simulink library "tqen"  (Simulink 8.2)
settings: Solver=ode45  SolverMode=SingleTasking  StartTime=0.0  StopTime=10.0  RelTol=1e-3
undefined symbols (not defined in the file or in its folder): ATQEN_BaseBrkDerateRatD_X_pct, ATQEN_BaseVehSpdRatD_X_kph, ATQEN_CruzAccLimIMult_X_mps2, ATQEN_CruzAccLimPMult_X_mps2, ATQEN_CruzContIMult_X_kph, ATQEN_CruzContPMult_X_kph, ATQEN_EngTqBrkMap_X_erpm, C_TASK_5MS_S, C_TICK_TIME_S, ENUM_ECMTQSOURCE_EXTERNAL, ENUM_ECMTQSOURCE_INTERNAL, ENUM_ECMTQSOURCE_TORQUELIM, ENUM_EMSHYBRIDOPSTATE_HYBRIDENABLE, ENUM_EMSOPSTATE_NORMAL, ENUM_GEARPOSN_PN, FALSE, KTQEN_AccelPedalFiltTm_s, KTQEN_BrakeSWTqDsblTimeThres_s, KTQEN_CruzAccLimErrGain_rat, KTQEN_CruzAccLimIGain_rat, KTQEN_CruzAccLimIMax_Nm, KTQEN_CruzAccLimIMin_Nm, KTQEN_CruzAccLimIRest_flg, KTQEN_CruzAccLimPGain_rat, KTQEN_CruzContAccLim_G, KTQEN_CruzContAccLimTqMax_Nm, KTQEN_CruzContAccLimTqMin_Nm, KTQEN_CruzContEnblSW_flg, KTQEN_CruzContErrGain_rat, KTQEN_CruzContIGain_rat, KTQEN_CruzContIMax_Nm, KTQEN_CruzContIMin_Nm, KTQEN_CruzContIRest_flg, KTQEN_CruzContPGain_rat, KTQEN_CruzContResumeSW_flg, KTQEN_CruzContSetSW_flg, KTQEN_CruzDsblDefaultTq_Nm, KTQEN_CruzSpdChgTimeThres_s, KTQEN_CruzTgSpdSetFalRate_kphps, KTQEN_CruzTgSpdSetRisRate_kphps, KTQEN_EngBrkTqMaxOvrd_Nm, KTQEN_EngBrkTqMinOvrd_Nm, KTQEN_VehAccCalRate_s, KTQEN_VehAccFltConst_s, KTQEN_VehSpdMaxVal_kph, KTQEN_VSGOVErrGain_rat, KTQEN_VSGOVIGain_rat, KTQEN_VSGOVIMax_Nm, KTQEN_VSGOVIMin_Nm, KTQEN_VSGOVIRest_flg, KTQEN_VSGOVMinVehSpd_kph, KTQEN_VSGOVPGain_rat, KTQEN_VSGOVTqDefault_Nm, KTQEN_VSGOVTqMax_Nm, KTQEN_VSGOVTqMin_Nm, MTQEN_BaseBrkDerateRatD_Y_pct, MTQEN_BasePedalSportMapHiSpdD_Z_pct, MTQEN_BasePedalSportMapLoSpdD_Z_pct, MTQEN_BaseTqSupptDeltPdlD_X_pctps, MTQEN_BaseTqSupptDeltPdlD_Y_pct ... (+9)
libraries: hcu_lib x6, tqen x3, simulink x1
(part 1 of 2)
settings Model: Creator=13192  LastModifiedBy=14069

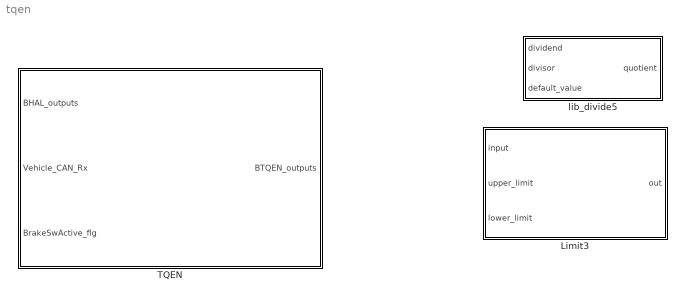
== system tqen ==
  Limit3 : Subsystem
      mask Display: disp('Limitation')
  TQEN : Subsystem
      settings: RTWSystemCode=Nonreusable function  RTWFcnNameOpts=Use subsystem name  RTWFileNameOpts=Use subsystem name
  lib_divide5 : Subsystem  RTWFcnName=plaus_check  mask(divide){}
      mask help: Performs a division operation. If the divisor is found to be between -0.00001 and +0.00001 then a failsafe value is passed to the output.
      mask Display: disp('Divide\nTQM');

== system tqen/Limit3 ==
  input : Inport
  upper_limit : Inport  Port=2
  lower_limit : Inport  Port=3
  MinMax10 : MinMax  Function=max  Inputs=2
  MinMax5 : MinMax  Inputs=2
  out : Outport
  wires:
  lower_limit/1 -> MinMax10/2
  upper_limit/1 -> MinMax5/2
  MinMax10/1 -> out/1
  input/1 -> MinMax5/1
  MinMax5/1 -> MinMax10/1

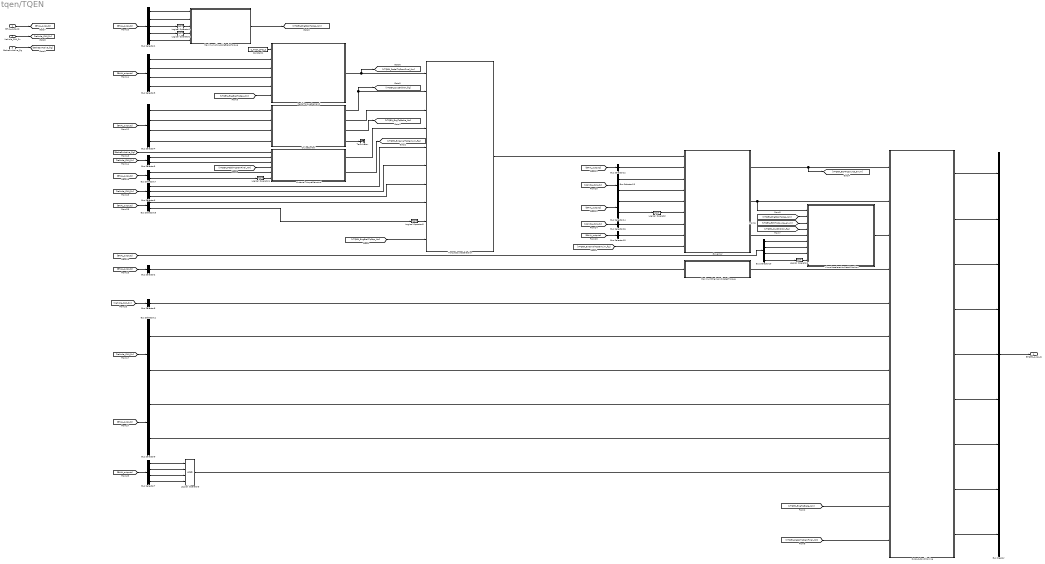
== system tqen/TQEN ==
  BHAL_outputs : Inport  OutDataTypeStr=Bus: BHAL_outputs
  Vehicle_CAN_Rx : Inport  Port=2
  BrakeSwActive_flg : Inport  Port=3
  Bus Creator : BusCreator  Inputs=9  OutDataTypeStr=Bus: BTQEN_outputs
  Bus Selector1 : BusSelector  OutputSignals=VHAL_EngTqMax_Nm,VHAL_EngTqMin_Nm,VHAL_EngTqMinInvalid_flg,VHAL_EngTqMaxInvalid_flg,VHAL_EngSpd_erpm
  Bus Selector10 : BusSelector  OutputSignals=VHAL_EngSpd_erpm,VHAL_AccelPedalPosn_pct,VHAL_EngTqMin_Nm,VHAL_EngTqMinInvalid_flg
  Bus Selector11 : BusSelector  OutputSignals=ADAS2.ADAS_PTTqReq,ADAS2.ADAS_PTTqReq_A
  Bus Selector12 : BusSelector  OutputSignals=VHAL_VehSpd_kph
  Bus Selector13 : BusSelector  OutputSignals=ADAS3.ADAS_VehSpdLim,ADAS3.ADAS_VehSpdLim_A
  Bus Selector14 : BusSelector  OutputSignals=VHAL_NowGearPosn_enum,VHAL_VehSpdInvalid_flg
  Bus Selector15 : BusSelector  OutputSignals=VHAL_BrkLampOn_flg
  Bus Selector16 : BusSelector  OutputSignals=ADAS2.ADAS_PTTqReq_A
  Bus Selector17 : BusSelector  OutputSignals=VHAL_EngTqMin_Nm,VHAL_EngTqMinInvalid_flg
  Bus Selector18 : BusSelector  OutputSignals=VHAL_EngTqMin_Nm,VHAL_EngTqMinInvalid_flg
  Bus Selector2 : BusSelector  OutputSignals=VHAL_EngTqFriction_Nm
  Bus Selector3 : BusSelector  OutputSignals=VHAL_AccelPedalPosn_pct,VHAL_BrkLampOn_flg,VHAL_EngSpd_erpm,VHAL_VehSpd_kph
  Bus Selector4 : BusSelector  OutputSignals=VHAL_BrkLampOn_flg,VHAL_VehSpd_kph,VHAL_EngTqIndicatedCOR_Nm,VHAL_EngTqFriction_Nm
  Bus Selector5 : BusSelector  OutputSignals=ADAS2.ADAS_PTTqReq,ADAS2.ADAS_PTTqReq_A
  Bus Selector6 : BusSelector  OutputSignals=ADAS2.ADAS_PTTqReq_A,ADAS2.ADAS_ForceIdle,ADAS2.ADAS_ForceIdle_A
  Bus Selector7 : BusSelector  OutputSignals=VHAL_CANMsgValidECM1_flg,VHAL_CANMsgValidECM2_flg,VHAL_CANMsgValidECM3_flg,VHAL_CANMsgValidECM9_flg
  Bus Selector8 : BusSelector  OutputSignals=ECM1.CAN_TQ_STND
  Bus Selector9 : BusSelector  OutputSignals=VHAL_EMSHybridOpState_enum,VHAL_EMSOpState_enum
  Constant1 : Constant  Value=C_TASK_5MS_S  OutDataTypeStr=single
  CruiseControl : Subsystem  TreatAsAtomicUnit=on
  ExternalTorqueDemand : Subsystem
  Governor : Subsystem
  Logical Operator{,1..2,4..6} (6 alike) : Logic  Operator=NOT  AllPortsSameDT=off  OutDataTypeStr=boolean
  Logical Operator3 : Logic  Inputs=4  AllPortsSameDT=off  OutDataTypeStr=boolean
  MaximumAllowableBrakeTorque : Subsystem
  MaximumEngineIndicatedTorque : Subsystem
  Output_Conditioning : Subsystem
  PedalTorqueDemand : Subsystem
  Terminator : Terminator
  TorqueSourceSelection : Subsystem
  VirtualAccelerationPedalPosition : Subsystem
  BTQEN_outputs : Outport  OutDataTypeStr=Bus: BTQEN_outputs
  wires:
  Logical Operator6/1 -> VirtualAccelerationPedalPosition/9(VDINR_EngTqMinValid_flg)
  Bus Selector10/4 -> Logical Operator6/1  "<VHAL_EngTqMinInvalid_flg>"
  Bus Selector10/3 -> VirtualAccelerationPedalPosition/8(VDINR_EngTqMin_Nm)  "<VHAL_EngTqMin_Nm>"
  Logical Operator5/1 -> TorqueSourceSelection/9(VDINR_EngTqMinValid_flg)
  [BHAL_outputs] -> Bus Selector18/1
  Bus Selector18/2 -> Logical Operator5/1  "<VHAL_EngTqMinInvalid_flg>"
  Bus Selector18/1 -> TorqueSourceSelection/8(VDINR_EngTqMin_Nm)  "<VHAL_EngTqMin_Nm>"
  Logical Operator4/1 -> ExternalTorqueDemand/6(VDINR_EngTqMinValid_flg)
  [BHAL_outputs] -> Bus Selector17/1
  Bus Selector17/2 -> Logical Operator4/1  "<VHAL_EngTqMinInvalid_flg>"
  Bus Selector17/1 -> ExternalTorqueDemand/5(VDINR_EngTqMin_Nm)  "<VHAL_EngTqMin_Nm>"
  [BHAL_outputs] -> Bus Selector9/1
  Logical Operator3/1 -> Output_Conditioning/10(VDINR_ECMCANValid_flg)
  Bus Selector7/2 -> Logical Operator3/2  "<VHAL_CANMsgValidECM2_flg>"
  Bus Selector7/4 -> Logical Operator3/4  "<VHAL_CANMsgValidECM9_flg>"
  Bus Selector7/3 -> Logical Operator3/3  "<VHAL_CANMsgValidECM3_flg>"
  Bus Selector7/1 -> Logical Operator3/1  "<VHAL_CANMsgValidECM1_flg>"
  [BHAL_outputs] -> Bus Selector7/1
  Bus Selector15/1 -> Governor/8(VDINR_BrkLampOn_flg)  "<VHAL_BrkLampOn_flg>"
  Bus Selector16/1 -> Governor/7(VDINR_ADASPTTqReqApplable_flg)  "<ADAS_PTTqReq_A>"
  [Vehicle_CAN_Rx] -> Bus Selector16/1
  [BHAL_outputs] -> Bus Selector15/1
  Bus Selector14/2 -> Logical Operator/1  "<VHAL_VehSpdInvalid_flg>"
  Bus Selector14/1 -> Governor/5(VDINR_NowGearPosn_enum)  "<VHAL_NowGearPosn_enum>"
  Bus Selector13/2 -> Governor/4(VDINR_ADASVehSpdLimReqValid_flg)  "<ADAS_VehSpdLim_A>"
  Bus Selector13/1 -> Governor/3(VDINR_ADASVehSpdLimReq_kph)  "<ADAS_VehSpdLim>"
  [BHAL_outputs] -> Bus Selector14/1
  [VTQEN_PedalTqDemFinal_Nm] -> ExternalTorqueDemand/4(VTQEN_PedalTqDemFinal_Nm)
  Output_Conditioning/9("VTQEN_PedalTqDemFinal_Nm ") -> Bus Creator/9
  [VTQEN_PedalTqDemFinal_Nm] -> Output_Conditioning/12(VTQEN_PedalTqDemFinal_Nm)
  Bus Selector6/3 -> TorqueSourceSelection/7(VDINR_ADASPTIdleReqValid_flg)  "<ADAS_ForceIdle_A>"
  Bus Selector6/2 -> TorqueSourceSelection/6(VDINR_ADASPTIdleReq_flg)  "<ADAS_ForceIdle>"
  Output_Conditioning/3("VTQEN_FinalAccelPedalPosn_pct ") -> Bus Creator/3
  Bus Selector10/2 -> VirtualAccelerationPedalPosition/7(VDINR_HWAccelPedalPosn_pct)  "<VHAL_AccelPedalPosn_pct>"
  Bus Selector10/1 -> VirtualAccelerationPedalPosition/6(VDINR_EngSpd_erpm)  "<VHAL_EngSpd_erpm>"
  [VTQEN_CruzEnblOn_flg] -> VirtualAccelerationPedalPosition/4(VTQEN_CruzEnblOn_flg)
  [VTQEN_ECMTqSource_enum] -> VirtualAccelerationPedalPosition/3(VTQEN_ECMTqSource_enum)
  [VTQEN_EngBrakTqCap_Nm] -> VirtualAccelerationPedalPosition/2(VTQEN_EngBrakTqCap_Nm)
  Governor/3(VTQEN_VSGOVOn_flg) -> VirtualAccelerationPedalPosition/5(VTQEN_VSGOVOn_flg)
  VirtualAccelerationPedalPosition/1(VTQEN_FinalAccelPedalPosn_pct) -> Output_Conditioning/3(VTQEN_FinalAccelPedalPosn_pct)
  [VTQEN_ExternalTqDemLim_flg] -> Governor/9(VTQEN_ExternalTqDemLim_flg)
  ExternalTorqueDemand/2(VTQEN_ExternalTqDemLim_flg) -> [VTQEN_ExternalTqDemLim_flg]
  Output_Conditioning/8("VTQEN_EngTqBrake_Nm ") -> Bus Creator/8
  Output_Conditioning/7(VTQEN_ECMExtnTqAvailable_flg) -> Bus Creator/7
  Output_Conditioning/6(VTQEN_AckCurPTTqReqApplable_flg) -> Bus Creator/6
  Output_Conditioning/5(VTQEN_AckCurPTTqReq_Nm) -> Bus Creator/5
  Bus Selector11/2 -> Output_Conditioning/7(VDINR_ADASPTTqReqApplable_flg)  "<ADAS_PTTqReq_A>"
  Bus Selector11/1 -> Output_Conditioning/6(VDINR_ADASPTTqReq_Nm)  "<ADAS_PTTqReq>"
  [VTQEN_EngTqBrake_Nm] -> Output_Conditioning/11(VTQEN_EngTqBrake_Nm)
  Output_Conditioning/1("VTQEN_ECMTqSource_enum ") -> Bus Creator/1
  CruiseControl/3(VTQEN_EngTqBrake_Nm) -> [VTQEN_EngTqBrake_Nm]
  Logical Operator/1 -> Governor/6(VDINR_VehSpdValid_flg)
  Governor/1(VTQEN_ECMTqSource_enum) -> [VTQEN_ECMTqSource_enum], Output_Conditioning/1(VTQEN_ECMTqSource_enum)
  Output_Conditioning/4(VTQEN_EngIndTqReqMax_pct) -> Bus Creator/4
  Output_Conditioning/2(VTQEN_EngBrakTqReqFinal_Nm) -> Bus Creator/2
  Governor/2(VTQEN_EngBrakTqReqFinal_Nm) -> VirtualAccelerationPedalPosition/1(VTQEN_EngBrakTqReqFinal_Nm), Output_Conditioning/2("VTQEN_EngBrakTqReqFinal_Nm ")
  MaximumEngineIndicatedTorque/1(VTQEN_EngIndTqReqMax_Nm) -> Output_Conditioning/4(VTQEN_EngIndTqReqMax_Nm)
  ExternalTorqueDemand/1(VTQEN_ExternalTqDem_Nm) -> TorqueSourceSelection/4(VTQEN_ExternalTqDem_Nm)
  CruiseControl/2(VTQEN_CruzContTqComdFinal_Nm) -> TorqueSourceSelection/3(VTQEN_CruzContTqComdFinal_Nm)
  CruiseControl/1(VTQEN_CruzEnblOn_flg) -> [VTQEN_CruzEnblOn_flg], TorqueSourceSelection/2(VTQEN_CruzEnblOn_flg)
  Bus Selector6/1 -> TorqueSourceSelection/5(VDINR_ADASPTTqReqApplable_flg)  "<ADAS_PTTqReq_A>"
  CruiseControl/4(VTQEN_CruzStandby_flg) -> Terminator/1
  Bus Selector4/4 -> CruiseControl/4(VDINR_EngTqFriction_Nm)  "<VHAL_EngTqFriction_Nm>"
  Bus Selector4/3 -> CruiseControl/3(VDINR_EngTqIndicatedCOR_Nm)  "<VHAL_EngTqIndicatedCOR_Nm>"
  Bus Selector4/2 -> CruiseControl/2(VDINR_VehSpd_kph)  "<VHAL_VehSpd_kph>"
  Bus Selector4/1 -> CruiseControl/1(VDINR_BrkLampOn_flg)  "<VHAL_BrkLampOn_flg>"
  [VTQEN_EngBrakTqCap_Nm] -> TorqueSourceSelection/10(VTQEN_EngBrakTqCap_Nm)
  [VTQEN_EngBrakTqCap_Nm] -> PedalTorqueDemand/6(VTQEN_EngBrakTqCap_Nm)
  Bus Creator/1 -> BTQEN_outputs/1  "BTQEN_outputs"
  [BHAL_outputs] -> Bus Selector1/1
  TorqueSourceSelection/1(VTQEN_EngBrakTqReqRaw_Nm) -> Governor/1(VTQEN_EngBrakTqReqRaw_Nm)
  MaximumAllowableBrakeTorque/1(VTQEN_EngBrakTqCap_Nm) -> [VTQEN_EngBrakTqCap_Nm]
  PedalTorqueDemand/1(VTQEN_PedalTqDemFinal_Nm) -> [VTQEN_PedalTqDemFinal_Nm], TorqueSourceSelection/1(VTQEN_PedalTqDemFinal_Nm)
  Bus Selector1/1 -> MaximumAllowableBrakeTorque/1(VDINR_EngTqMax_Nm)  "<VHAL_EngTqMax_Nm>"
  Bus Selector1/2 -> MaximumAllowableBrakeTorque/2(VDINR_EngTqMin_Nm)  "<VHAL_EngTqMin_Nm>"
  Bus Selector1/3 -> Logical Operator1/1  "<VHAL_EngTqMinInvalid_flg>"
  Bus Selector1/4 -> Logical Operator2/1  "<VHAL_EngTqMaxInvalid_flg>"
  Bus Selector1/5 -> MaximumAllowableBrakeTorque/5(VDINR_EngSpd_erpm)  "<VHAL_EngSpd_erpm>"
  Constant1/1 -> PedalTorqueDemand/1(task_time_s)
  Bus Selector8/1 -> Output_Conditioning/5(VDINR_StandardTq_Nm)  "<CAN_TQ_STND>"
  Bus Selector2/1 -> MaximumEngineIndicatedTorque/1(VDINR_EngTqFriction_Nm)  "<VHAL_EngTqFriction_Nm>"
  Logical Operator1/1 -> MaximumAllowableBrakeTorque/3(VDINR_EngTqMinValid_flg)
  Logical Operator2/1 -> MaximumAllowableBrakeTorque/4(VDINR_EngTqMaxValid_flg)
  Bus Selector3/4 -> PedalTorqueDemand/5(VDINR_VehSpd_kph)  "<VHAL_VehSpd_kph>"
  Bus Selector3/1 -> PedalTorqueDemand/2(VDINR_HWAccelPedalPosn_pct)  "<VHAL_AccelPedalPosn_pct>"
  Bus Selector3/2 -> PedalTorqueDemand/3(VDINR_BrkLampOn_flg)  "<VHAL_BrkLampOn_flg>"
  Bus Selector3/3 -> PedalTorqueDemand/4(VDINR_EngSpd_erpm)  "<VHAL_EngSpd_erpm>"
  [BrakeSwActive_flg] -> ExternalTorqueDemand/1(VDINR_BrakeSwActive_flg)
  [Vehicle_CAN_Rx] -> Bus Selector5/1
  Bus Selector5/2 -> ExternalTorqueDemand/3(VDINR_ADASPTTqReqValid_flg)  "<ADAS_PTTqReq_A>"
  Bus Selector5/1 -> ExternalTorqueDemand/2(VDINR_ADASPTTqReq_Nm)  "<ADAS_PTTqReq>"
  BHAL_outputs/1 -> [BHAL_outputs]
  Vehicle_CAN_Rx/1 -> [Vehicle_CAN_Rx]
  BrakeSwActive_flg/1 -> [BrakeSwActive_flg]
  [BHAL_outputs] -> Bus Selector3/1
  [BHAL_outputs] -> Bus Selector4/1
  [Vehicle_CAN_Rx] -> Bus Selector6/1
  [BHAL_outputs] -> Bus Selector2/1
  [Vehicle_CAN_Rx] -> Bus Selector11/1
  Bus Selector9/1 -> Output_Conditioning/8(VDINR_EMSHybridOpState_enum)  "<VHAL_EMSHybridOpState_enum>"
  Bus Selector9/2 -> Output_Conditioning/9(VDINR_EMSOpState_enum)  "<VHAL_EMSOpState_enum>"
  [Vehicle_CAN_Rx] -> Bus Selector8/1
  [BHAL_outputs] -> Bus Selector10/1
  [BHAL_outputs] -> Bus Selector12/1
  Bus Selector12/1 -> Governor/2(VDINR_VehSpd_kph)  "<VHAL_VehSpd_kph>"
  [Vehicle_CAN_Rx] -> Bus Selector13/1

== system tqen/lib_divide5 ==
  dividend : Inport
  divisor : Inport  Port=2
  default_value : Inport  Port=3
  Divide : Product  Inputs=*/
  Inter_Test : Subsystem  mask(Interval Test){IntervalClosedRight=on, uplimit=0.00001, IntervalClosedLeft=on, lowlimit=-0.00001, LogicOutDataTypeMode=boolean}
      mask prompts: IntervalClosedRight "Interval closed on right"; uplimit "Upper limit:"; IntervalClosedLeft "Interval closed on left"; lowlimit "Lower limit:"; LogicOutDataTypeMode "Output data type mode:"
      mask help: If the input is in the interval between the lower limit and the upper limit, then the output is TRUE, otherwise it is FALSE.
      mask init:
      | if IntervalClosedLeft
      |   lOff = 0;
      |   lRelop = '<=';
      | else
      |   lOff = 0.1;
      |   lRelop = '<';
      | end
      | if IntervalClosedRight
      |   rOff = 0;
      |   uRelop = '<=';
      | else
      |   rOff = 0.1;
      |   uRelop = '<';
      | end
      | 
      | blkH = gcbh;
      | blkName = getfullname(blkH);
      | 
      | set_param([blkName,'/Upper_Test'],'relop',uRelop);
      | set_param([blkName,'/Lower_Test'],'relop',lRelop);
      | if strcmp(get_param(blkH,'LogicOutDataTypeMode'),'boolean')
      | set_param([blkName,'/AND'],'OutDataTypeMode','Boolean');
      | else
      | set_param([blkName,'/AND'],'OutDataTypeMode','Specify via dialog');
      | end
      mask TypeOptions LogicOutDataTypeMode: uint8 | boolean
      mask Display: plot([0 1],[0.3 0.3],[0.3 0.3],[0 1],[0 0.2 0.2],[0.35 0.35 0.55-lOff],[0.2 0.2 0.55 0.55],[0.55+lOff 0.75 0.75 0.55+rOff],[0.55 0.55 1],[0.55-rOff 0.35 0.35]);
  Logical_Operator : Logic  Operator=NOT  AllPortsSameDT=off  OutDataTypeStr=boolean
  Switch : Switch  Criteria=u2 ~= 0  Threshold=0.5
  quotient : Outport
  wires:
  divisor/1 -> Inter_Test/1(u), Divide/2
  dividend/1 -> Divide/1
  Divide/1 -> Switch/1
  Switch/1 -> quotient/1
  Inter_Test/1(y) -> Logical_Operator/1
  default_value/1 -> Switch/3
  Logical_Operator/1 -> Switch/2

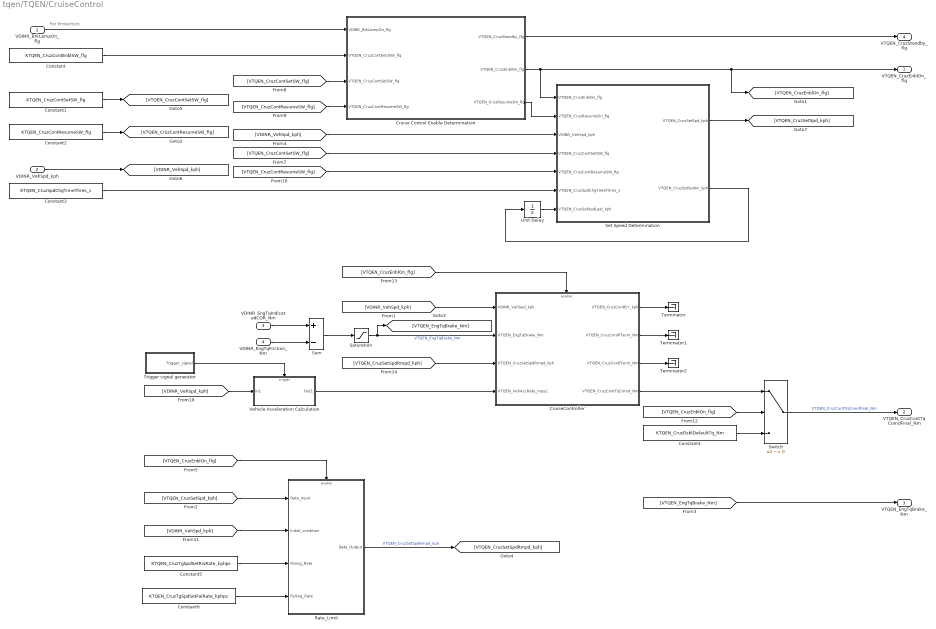
== system tqen/TQEN/CruiseControl ==
  note: For Protection
  VDINR_BrkLampOn_flg : Inport
  VDINR_VehSpd_kph : Inport  Port=2
  VDINR_EngTqIndicatedCOR_Nm : Inport  Port=3
  VDINR_EngTqFriction_Nm : Inport  Port=4
  Constant : Constant  Value=KTQEN_CruzContEnblSW_flg
  Constant1 : Constant  Value=KTQEN_CruzContSetSW_flg
  Constant2 : Constant  Value=KTQEN_CruzContResumeSW_flg
  Constant3 : Constant  Value=KTQEN_CruzSpdChgTimeThres_s
  Constant4 : Constant  Value=KTQEN_CruzDsblDefaultTq_Nm
  Constant5 : Constant  Value=KTQEN_CruzTgSpdSetRisRate_kphps
  Constant6 : Constant  Value=KTQEN_CruzTgSpdSetFalRate_kphps
  Cruise Control Enable Determination : Stateflow chart  TreatAsAtomicUnit=on
  CruiseController : Subsystem  TreatAsAtomicUnit=on
  Rate_Limit : Subsystem  TreatAsAtomicUnit=on
  Saturation : Saturate  UpperLimit=inf  LowerLimit=0
  Set Speed Determination : Stateflow chart  TreatAsAtomicUnit=on
  Sum : Sum  Inputs=+-
  Switch : Switch  Criteria=u2 ~= 0
  Terminator : Terminator
  Terminator1 : Terminator
  Terminator2 : Terminator
  Trigger signal generator : Subsystem  TreatAsAtomicUnit=on
  Unit Delay : UnitDelay  SampleTime=-1
  Vehicle Acceleration Calculation : Subsystem
  VTQEN_CruzEnblOn_flg : Outport
  VTQEN_CruzContTqComdFinal_Nm : Outport  Port=2
  VTQEN_EngTqBrake_Nm : Outport  Port=3
  VTQEN_CruzStandby_flg : Outport  Port=4
  wires:
  [VTQEN_EngTqBrake_Nm] -> VTQEN_EngTqBrake_Nm/1
  [VDINR_VehSpd_kph] -> Vehicle Acceleration Calculation/1(In1)
  Trigger signal generator/1(Trigger_signal) -> Vehicle Acceleration Calculation/Trigger
  Rate_Limit/1(Data_Output) -> [VTQEN_CruzSetSpdRmpd_kph]  "VTQEN_CruzSetSpdRmpd_kph"
  Saturation/1 -> [VTQEN_EngTqBrake_Nm], CruiseController/2(VTQEN_EngTqBrake_Nm)  "VTQEN_EngTqBrake_Nm"
  Sum/1 -> Saturation/1
  VDINR_EngTqFriction_Nm/1 -> Sum/2
  VDINR_EngTqIndicatedCOR_Nm/1 -> Sum/1
  [VTQEN_CruzEnblOn_flg] -> Rate_Limit/Enable
  [VTQEN_CruzEnblOn_flg] -> CruiseController/Enable
  Constant3/1 -> Set Speed Determination/6(VTQEN_CruzSpdChgTimeThres_s)
  Cruise Control Enable Determination/1(VTQEN_CruzStandby_flg) -> VTQEN_CruzStandby_flg/1
  Constant2/1 -> [VTQEN_CruzContResumeSW_flg]
  Constant1/1 -> [VTQEN_CruzContSetSW_flg]
  Constant/1 -> Cruise Control Enable Determination/2(VTQEN_CruzContEnblSW_flg)
  Set Speed Determination/1(VTQEN_CruzSetSpd_kph) -> [VTQEN_CruzSetSpd_kph]
  Unit Delay/1 -> Set Speed Determination/7(VTQEN_CruzSetSpdLast_kph)
  Set Speed Determination/2(VTQEN_CruzSetSpdIni_kph) -> Unit Delay/1
  [VDINR_VehSpd_kph] -> Set Speed Determination/3(VDINR_VehSpd_kph)
  [VTQEN_CruzContResumeSW_flg] -> Set Speed Determination/5(VTQEN_CruzContResumeSW_flg)
  [VTQEN_CruzContSetSW_flg] -> Set Speed Determination/4(VTQEN_CruzContSetSW_flg)
  [VTQEN_CruzContResumeSW_flg] -> Cruise Control Enable Determination/4(VTQEN_CruzContResumeSW_flg)
  [VTQEN_CruzContSetSW_flg] -> Cruise Control Enable Determination/3(VTQEN_CruzContSetSW_flg)
  VDINR_BrkLampOn_flg/1 -> Cruise Control Enable Determination/1(VDINR_BrkLampOn_flg)
  Cruise Control Enable Determination/3(VTQEN_CruzResumeOn_flg) -> Set Speed Determination/2(VTQEN_CruzResumeOn_flg)
  Cruise Control Enable Determination/2(VTQEN_CruzEnblOn_flg) -> VTQEN_CruzEnblOn_flg/1, [VTQEN_CruzEnblOn_flg], Set Speed Determination/1(VTQEN_CruzEnblOn_flg)
  Constant6/1 -> Rate_Limit/4(Falling_Rate)
  Constant5/1 -> Rate_Limit/3(Rising_Rate)
  [VDINR_VehSpd_kph] -> Rate_Limit/2(Initial_condition)
  [VTQEN_CruzSetSpd_kph] -> Rate_Limit/1(Data_Input)
  Vehicle Acceleration Calculation/1(Out1) -> CruiseController/4(VTQEN_VehAccRate_mps2)
  CruiseController/3(VTQEN_CruzContITerm_Nm) -> Terminator2/1
  CruiseController/2(VTQEN_CruzContPTerm_Nm) -> Terminator1/1
  CruiseController/1(VTQEN_CruzContErr_kph) -> Terminator/1
  Switch/1 -> VTQEN_CruzContTqComdFinal_Nm/1  "VTQEN_CruzContTqComdFinal_Nm"
  [VTQEN_CruzSetSpdRmpd_kph] -> CruiseController/3(VTQEN_CruzSetSpdRmpd_kph)
  [VDINR_VehSpd_kph] -> CruiseController/1(VDINR_VehSpd_kph)
  CruiseController/4(VTQEN_CruzContTqComd_Nm) -> Switch/1
  Constant4/1 -> Switch/3
  [VTQEN_CruzEnblOn_flg] -> Switch/2
  VDINR_VehSpd_kph/1 -> [VDINR_VehSpd_kph]

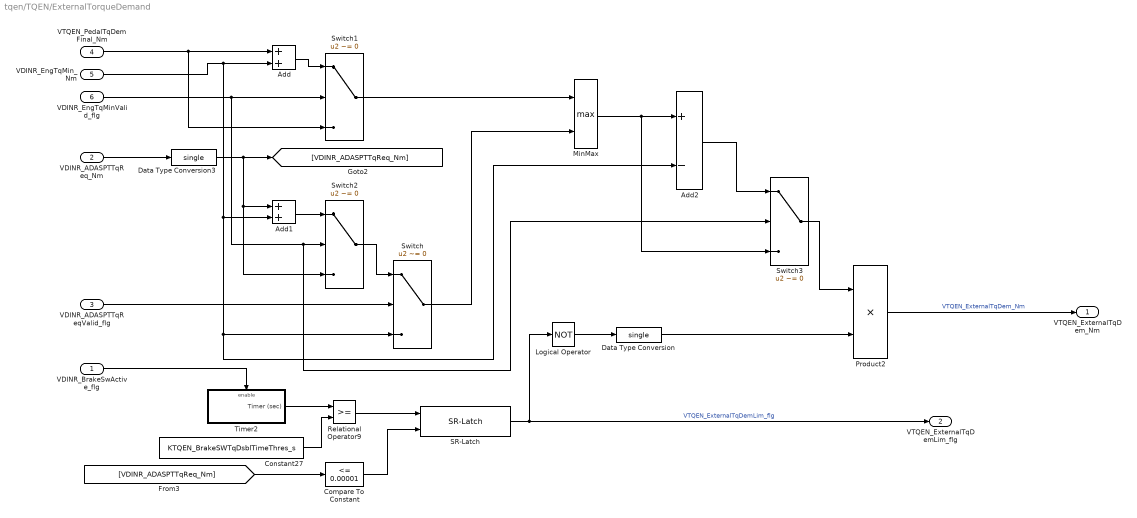
== system tqen/TQEN/ExternalTorqueDemand ==
  VDINR_BrakeSwActive_flg : Inport
  VDINR_ADASPTTqReq_Nm : Inport  Port=2
  VDINR_ADASPTTqReqValid_flg : Inport  Port=3
  VTQEN_PedalTqDemFinal_Nm : Inport  Port=4
  VDINR_EngTqMin_Nm : Inport  Port=5
  VDINR_EngTqMinValid_flg : Inport  Port=6
  Add : Sum
  Add1 : Sum
  Add2 : Sum  Inputs=+-
  Compare To Constant : simulink/Logic and Bit Operations/Compare To Constant  relop=<=  const=0.00001  OutDataTypeStr=boolean
  Constant27 : Constant  Value=KTQEN_BrakeSWTqDsblTimeThres_s
  Data Type Conversion : DataTypeConversion  OutDataTypeStr=single
  Data Type Conversion3 : DataTypeConversion  OutDataTypeStr=single
  Logical Operator : Logic  Operator=NOT  AllPortsSameDT=off  OutDataTypeStr=boolean
  MinMax : MinMax  Function=max  Inputs=2
  Product2 : Product  RndMeth=Zero
  Relational Operator9 : RelationalOperator  OutDataTypeStr=boolean
  SR-Latch : hcu_lib/SR-Latch  SystemSampleTime=-1
  Switch{,1..3} (4 alike) : Switch  Criteria=u2 ~= 0
  Timer2 : Subsystem  TreatAsAtomicUnit=on
  VTQEN_ExternalTqDem_Nm : Outport
  VTQEN_ExternalTqDemLim_flg : Outport  Port=2
  wires:
  Data Type Conversion3/1 -> Switch2/3, Add1/1, [VDINR_ADASPTTqReq_Nm]
  Add/1 -> Switch1/1
  VDINR_EngTqMinValid_flg/1 -> Switch3/2, Switch2/2, Switch1/2
  Switch3/1 -> Product2/1
  Switch1/1 -> MinMax/1
  VTQEN_PedalTqDemFinal_Nm/1 -> Add/1, Switch1/3
  [VDINR_ADASPTTqReq_Nm] -> Compare To Constant/1
  Compare To Constant/1 -> SR-Latch/2
  Relational Operator9/1 -> SR-Latch/1
  SR-Latch/1 -> VTQEN_ExternalTqDemLim_flg/1, Logical Operator/1  "VTQEN_ExternalTqDemLim_flg"
  Logical Operator/1 -> Data Type Conversion/1
  Constant27/1 -> Relational Operator9/2
  Timer2/1(Timer (sec)) -> Relational Operator9/1
  Switch/1 -> MinMax/2
  VDINR_ADASPTTqReqValid_flg/1 -> Switch/2
  Product2/1 -> VTQEN_ExternalTqDem_Nm/1  "VTQEN_ExternalTqDem_Nm"
  Data Type Conversion/1 -> Product2/2
  VDINR_BrakeSwActive_flg/1 -> Timer2/Enable
  VDINR_ADASPTTqReq_Nm/1 -> Data Type Conversion3/1
  Switch2/1 -> Switch/1
  Add1/1 -> Switch2/1
  MinMax/1 -> Switch3/3, Add2/1
  Add2/1 -> Switch3/1
  VDINR_EngTqMin_Nm/1 -> Add/2, Switch/3, Add2/2, Add1/2

== system tqen/TQEN/Governor ==
  VTQEN_EngBrakTqReqRaw_Nm : Inport
  VDINR_VehSpd_kph : Inport  Port=2
  VDINR_ADASVehSpdLimReq_kph : Inport  Port=3
  VDINR_ADASVehSpdLimReqValid_flg : Inport  Port=4
  VDINR_NowGearPosn_enum : Inport  Port=5
  VDINR_VehSpdValid_flg : Inport  Port=6
  VDINR_ADASPTTqReqApplable_flg : Inport  Port=7
  VDINR_BrkLampOn_flg : Inport  Port=8
  VTQEN_ExternalTqDemLim_flg : Inport  Port=9
  Governor : Subsystem  TreatAsAtomicUnit=on
  Max_Min_Brake_Torque : Subsystem
  MinMax1 : MinMax  Inputs=2
  TorqueSourceDetermination : Subsystem
  Torque_Limitation : Subsystem
  Unit Delay : UnitDelay  SampleTime=-1
  Vehcle Speed Governing : Subsystem  TreatAsAtomicUnit=on
  VTQEN_ECMTqSource_enum : Outport
  VTQEN_EngBrakTqReqFinal_Nm : Outport  Port=2
  VTQEN_VSGOVOn_flg : Outport  Port=3
  wires:
  VDINR_ADASVehSpdLimReqValid_flg/1 -> Governor/3(VDINR_ADASVehSpdLimReqValid_flg)
  VDINR_BrkLampOn_flg/1 -> TorqueSourceDetermination/4(VDINR_BrkLampOn_flg)
  VTQEN_ExternalTqDemLim_flg/1 -> TorqueSourceDetermination/5(VTQEN_ExternalTqDemLim_flg)
  Unit Delay/1 -> Vehcle Speed Governing/1(VTQEN_ECMTqSource_enum)
  [VTQEN_ECMTqSource_enum] -> Unit Delay/1
  TorqueSourceDetermination/1(VTQEN_ECMTqSource_enum) -> [VTQEN_ECMTqSource_enum], VTQEN_ECMTqSource_enum/1
  VDINR_ADASPTTqReqApplable_flg/1 -> TorqueSourceDetermination/3(VDINR_ADASPTTqReqApplable_flg)
  MinMax1/1 -> TorqueSourceDetermination/1(VTQEN_EngBrakTqReqGoverd_Nm), Torque_Limitation/3(VTQEN_EngBrakTqReqGoverd_Nm)  "VTQEN_EngBrakTqReqGoverd_Nm"
  [VTQEN_EngBrakTqReqRaw_Nm] -> MinMax1/1
  Governor/1(VTQEN_VSGOVTqBound_Nm) -> TorqueSourceDetermination/2(VTQEN_VSGOVTqBound_Nm), MinMax1/2
  [VDINR_VehSpd_kph] -> Governor/6(VDINR_VehSpd_kph)
  VDINR_VehSpdValid_flg/1 -> Governor/5(VDINR_VehSpdValid_flg)
  VDINR_NowGearPosn_enum/1 -> Governor/4(VDINR_NowGearPosn_enum)
  Vehcle Speed Governing/2(VTQEN_VSGOVTqComdFinal_Nm) -> Governor/2(VTQEN_VSGOVTqComdFinal_Nm)
  Vehcle Speed Governing/1(VTQEN_VSGOVOn_flg) -> VTQEN_VSGOVOn_flg/1, Governor/1(VTQEN_VSGOVOn_flg)
  VDINR_ADASVehSpdLimReq_kph/1 -> Vehcle Speed Governing/4(VDINR_ADASVehSpdLimReq_kph)
  VDINR_VehSpd_kph/1 -> [VDINR_VehSpd_kph], Vehcle Speed Governing/2(VDINR_VehSpd_kph)
  Max_Min_Brake_Torque/2(VTQEN_EngBrakTqReqMin_Nm) -> Torque_Limitation/2(VTQEN_EngBrakTqReqMin_Nm)
  Max_Min_Brake_Torque/1(VTQEN_EngBrkTqReqMax_Nm) -> Torque_Limitation/1(VTQEN_EngBrkTqReqMax_Nm)
  Torque_Limitation/1(VTQEN_EngBrakTqReqFinal_Nm) -> VTQEN_EngBrakTqReqFinal_Nm/1
  VTQEN_EngBrakTqReqRaw_Nm/1 -> [VTQEN_EngBrakTqReqRaw_Nm], Vehcle Speed Governing/3(VTQEN_EngBrakTqReqRaw_Nm)

== system tqen/TQEN/MaximumAllowableBrakeTorque ==
  VDINR_EngTqMax_Nm : Inport
  VDINR_EngTqMin_Nm : Inport  Port=2
  VDINR_EngTqMinValid_flg : Inport  Port=3
  VDINR_EngTqMaxValid_flg : Inport  Port=4
  VDINR_EngSpd_erpm : Inport  Port=5
  EngTqCapacity : Subsystem
  VTQEN_EngBrakTqCap_Nm : Outport
  wires:
  VDINR_EngSpd_erpm/1 -> EngTqCapacity/5(VDINR_EngSpd_erpm)
  VDINR_EngTqMaxValid_flg/1 -> EngTqCapacity/4(VDINR_EngTqMaxValid_flg)
  VDINR_EngTqMinValid_flg/1 -> EngTqCapacity/3(VDINR_EngTqMinValid_flg)
  VDINR_EngTqMin_Nm/1 -> EngTqCapacity/2(VDINR_EngTqMin_Nm)
  VDINR_EngTqMax_Nm/1 -> EngTqCapacity/1(VDINR_EngTqMax_Nm)
  EngTqCapacity/1(VTQEN_EngBrakTqCap_Nm) -> VTQEN_EngBrakTqCap_Nm/1

== system tqen/TQEN/MaximumEngineIndicatedTorque ==
  VDINR_EngTqFriction_Nm : Inport
  Max_Indicated_Torque : Subsystem
  VTQEN_EngIndTqReqMax_Nm : Outport
  wires:
  VDINR_EngTqFriction_Nm/1 -> Max_Indicated_Torque/1(VDINR_EngTqFriction_Nm)
  Max_Indicated_Torque/1(VTQEN_EngIndTqReqMax_Nm) -> VTQEN_EngIndTqReqMax_Nm/1

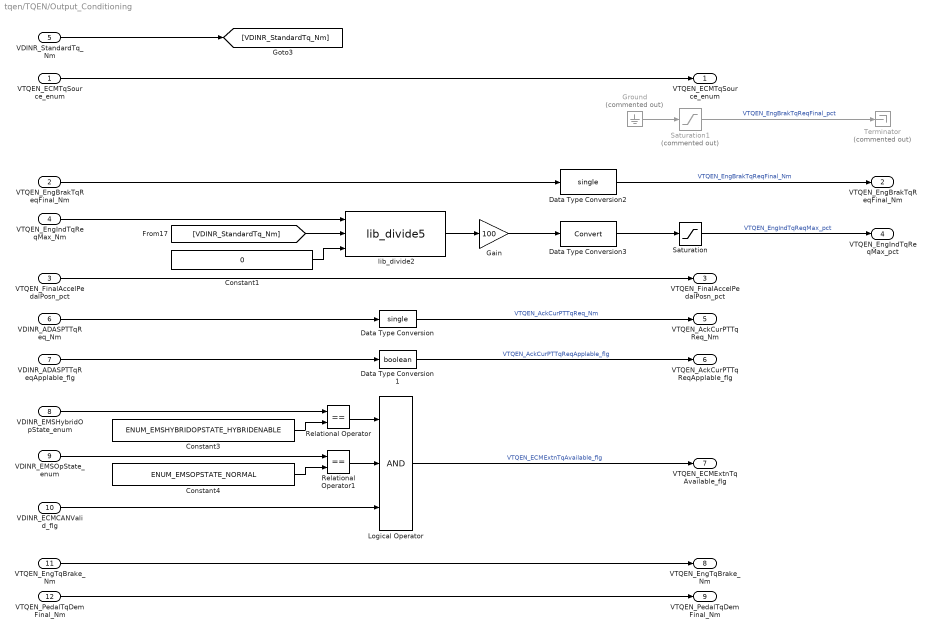
== system tqen/TQEN/Output_Conditioning ==
  VTQEN_ECMTqSource_enum : Inport
  "VTQEN_EngBrakTqReqFinal_Nm " : Inport  Port=2
  VTQEN_FinalAccelPedalPosn_pct : Inport  Port=3
  VTQEN_EngIndTqReqMax_Nm : Inport  Port=4
  VDINR_StandardTq_Nm : Inport  Port=5
  VDINR_ADASPTTqReq_Nm : Inport  Port=6
  VDINR_ADASPTTqReqApplable_flg : Inport  Port=7
  VDINR_EMSHybridOpState_enum : Inport  Port=8
  VDINR_EMSOpState_enum : Inport  Port=9
  VDINR_ECMCANValid_flg : Inport  Port=10
  VTQEN_EngTqBrake_Nm : Inport  Port=11
  VTQEN_PedalTqDemFinal_Nm : Inport  Port=12
  Constant1 : Constant  Value=0  OutDataTypeStr=single
  Constant3 : Constant  Value=ENUM_EMSHYBRIDOPSTATE_HYBRIDENABLE
  Constant4 : Constant  Value=ENUM_EMSOPSTATE_NORMAL
  Data Type Conversion : DataTypeConversion  OutDataTypeStr=single
  Data Type Conversion1 : DataTypeConversion  OutDataTypeStr=boolean
  Data Type Conversion2 : DataTypeConversion  OutDataTypeStr=single
  Data Type Conversion3 : DataTypeConversion
  Gain : Gain  Gain=100
  Ground : Ground  Commented=on
  Logical Operator : Logic  Inputs=3  AllPortsSameDT=off  OutDataTypeStr=boolean
  Relational Operator : RelationalOperator  Operator===  OutDataTypeStr=boolean
  Relational Operator1 : RelationalOperator  Operator===  OutDataTypeStr=boolean
  Saturation : Saturate  UpperLimit=100  LowerLimit=0
      settings: AttributesFormatString=lo=%<LowerLimit>\nup=%<UpperLimit>
  Saturation1 : Saturate  Commented=on  UpperLimit=100  LowerLimit=0
      settings: AttributesFormatString=lo=%<LowerLimit>\nup=%<UpperLimit>
  Terminator : Terminator  Commented=on
  lib_divide2 : tqen/lib_divide5
  "VTQEN_ECMTqSource_enum " : Outport
  VTQEN_EngBrakTqReqFinal_Nm : Outport  Port=2
  "VTQEN_FinalAccelPedalPosn_pct " : Outport  Port=3
  VTQEN_EngIndTqReqMax_pct : Outport  Port=4
  VTQEN_AckCurPTTqReq_Nm : Outport  Port=5
  VTQEN_AckCurPTTqReqApplable_flg : Outport  Port=6
  VTQEN_ECMExtnTqAvailable_flg : Outport  Port=7
  "VTQEN_EngTqBrake_Nm " : Outport  Port=8
  "VTQEN_PedalTqDemFinal_Nm " : Outport  Port=9
  wires:
  Data Type Conversion3/1 -> Saturation/1
  Data Type Conversion2/1 -> VTQEN_EngBrakTqReqFinal_Nm/1  "VTQEN_EngBrakTqReqFinal_Nm"
  VTQEN_PedalTqDemFinal_Nm/1 -> "VTQEN_PedalTqDemFinal_Nm "/1
  VTQEN_FinalAccelPedalPosn_pct/1 -> "VTQEN_FinalAccelPedalPosn_pct "/1
  Logical Operator/1 -> VTQEN_ECMExtnTqAvailable_flg/1  "VTQEN_ECMExtnTqAvailable_flg"
  VDINR_ECMCANValid_flg/1 -> Logical Operator/3
  Relational Operator1/1 -> Logical Operator/2
  Relational Operator/1 -> Logical Operator/1
  Constant4/1 -> Relational Operator1/2
  VDINR_EMSOpState_enum/1 -> Relational Operator1/1
  Constant3/1 -> Relational Operator/2
  VDINR_EMSHybridOpState_enum/1 -> Relational Operator/1
  VTQEN_EngTqBrake_Nm/1 -> "VTQEN_EngTqBrake_Nm "/1
  Data Type Conversion1/1 -> VTQEN_AckCurPTTqReqApplable_flg/1  "VTQEN_AckCurPTTqReqApplable_flg"
  VDINR_ADASPTTqReqApplable_flg/1 -> Data Type Conversion1/1
  Data Type Conversion/1 -> VTQEN_AckCurPTTqReq_Nm/1  "VTQEN_AckCurPTTqReq_Nm"
  VDINR_ADASPTTqReq_Nm/1 -> Data Type Conversion/1
  VTQEN_ECMTqSource_enum/1 -> "VTQEN_ECMTqSource_enum "/1
  VTQEN_EngIndTqReqMax_Nm/1 -> lib_divide2/1
  Constant1/1 -> lib_divide2/3
  lib_divide2/1 -> Gain/1
  Saturation/1 -> VTQEN_EngIndTqReqMax_pct/1  "VTQEN_EngIndTqReqMax_pct"
  Gain/1 -> Data Type Conversion3/1
  [VDINR_StandardTq_Nm] -> lib_divide2/2
  VDINR_StandardTq_Nm/1 -> [VDINR_StandardTq_Nm]
  Saturation1/1 -> Terminator/1  "VTQEN_EngBrakTqReqFinal_pct"
  Ground/1 -> Saturation1/1
  "VTQEN_EngBrakTqReqFinal_Nm "/1 -> Data Type Conversion2/1

== system tqen/TQEN/PedalTorqueDemand ==
  task_time_s : Inport
  VDINR_HWAccelPedalPosn_pct : Inport  Port=2
  VDINR_BrkLampOn_flg : Inport  Port=3
  VDINR_EngSpd_erpm : Inport  Port=4
  VDINR_VehSpd_kph : Inport  Port=5
  VTQEN_EngBrakTqCap_Nm : Inport  Port=6
  Gain : Gain  OutDataTypeStr=single
  PedalTorqueDemandCalculation : Subsystem
  VTQEN_PedalTqDemFinal_Nm : Outport
  wires:
  Gain/1 -> VTQEN_PedalTqDemFinal_Nm/1  "VTQEN_PedalTqDemFinal_Nm"
  PedalTorqueDemandCalculation/1(VTQEN_PedalTqDem_Nm) -> Gain/1
  VDINR_VehSpd_kph/1 -> PedalTorqueDemandCalculation/4(VDINR_VehSpd_kph)
  VDINR_EngSpd_erpm/1 -> PedalTorqueDemandCalculation/3(VDINR_EngSpd_erpm)
  VDINR_HWAccelPedalPosn_pct/1 -> PedalTorqueDemandCalculation/2(VDINR_HWAccelPedalPosn_pct)
  VTQEN_EngBrakTqCap_Nm/1 -> PedalTorqueDemandCalculation/6(VTQEN_EngBrakTqCap_Nm)
  VDINR_BrkLampOn_flg/1 -> PedalTorqueDemandCalculation/5(VDINR_BrkLampOn_flg)
  task_time_s/1 -> PedalTorqueDemandCalculation/1(task_time_s)

== system tqen/TQEN/TorqueSourceSelection ==
  VTQEN_PedalTqDemFinal_Nm : Inport
  VTQEN_CruzEnblOn_flg : Inport  Port=2
  VTQEN_CruzContTqComdFinal_Nm : Inport  Port=3
  VTQEN_ExternalTqDem_Nm : Inport  Port=4
  VDINR_ADASPTTqReqApplable_flg : Inport  Port=5
  VDINR_ADASPTIdleReq_flg : Inport  Port=6
  VDINR_ADASPTIdleReqValid_flg : Inport  Port=7
  VDINR_EngTqMin_Nm : Inport  Port=8
  VDINR_EngTqMinValid_flg : Inport  Port=9
  VTQEN_EngBrakTqCap_Nm : Inport  Port=10
  Add : Sum
  Add1 : Sum  Inputs=+-
  Constant : Constant  Value=single(60)
  Data Type Conversion : DataTypeConversion  OutDataTypeStr=single
  Divide : Product  Inputs=**
  Logical Operator : Logic  Operator=NOT  AllPortsSameDT=off  OutDataTypeStr=boolean
  Logical Operator1 : Logic  AllPortsSameDT=off  OutDataTypeStr=boolean
  MinMax : MinMax  Inputs=2
  Switch : Switch  Criteria=u2 ~= 0
  Switch1 : Switch  Criteria=u2 ~= 0
  Switch2 : Switch  Criteria=u2 ~= 0
  VTQEN_EngBrakTqReqRaw_Nm : Outport
  wires:
  Constant/1 -> Add1/2
  Add1/1 -> Switch2/3
  VDINR_EngTqMin_Nm/1 -> Add/2
  Divide/1 -> Add1/1, Add/1
  Add/1 -> Switch2/1
  Switch2/1 -> MinMax/1
  VDINR_EngTqMinValid_flg/1 -> Switch2/2
  Logical Operator1/1 -> Logical Operator/1
  VDINR_ADASPTIdleReqValid_flg/1 -> Logical Operator1/2
  Data Type Conversion/1 -> Divide/2
  Logical Operator/1 -> Data Type Conversion/1
  VDINR_ADASPTIdleReq_flg/1 -> Logical Operator1/1
  Switch/1 -> Divide/1  "VTQEN_EngBrakTqReqSel_Nm"
  VTQEN_CruzContTqComdFinal_Nm/1 -> Switch1/1
  VTQEN_CruzEnblOn_flg/1 -> [VTQEN_CruzEnblOn_flg], Switch1/2
  Switch1/1 -> Switch/3
  VTQEN_ExternalTqDem_Nm/1 -> Switch/1
  VDINR_ADASPTTqReqApplable_flg/1 -> [VDINR_ADASPTTqReqApplable_flg], Switch/2
  VTQEN_EngBrakTqCap_Nm/1 -> MinMax/2
  VTQEN_PedalTqDemFinal_Nm/1 -> Switch1/3
  MinMax/1 -> VTQEN_EngBrakTqReqRaw_Nm/1  "VTQEN_EngBrakTqReqRaw_Nm"

== system tqen/TQEN/VirtualAccelerationPedalPosition ==
  VTQEN_EngBrakTqReqFinal_Nm : Inport
  VTQEN_EngBrakTqCap_Nm : Inport  Port=2
  VTQEN_ECMTqSource_enum : Inport  Port=3
  VTQEN_CruzEnblOn_flg : Inport  Port=4
  VTQEN_VSGOVOn_flg : Inport  Port=5
  VDINR_EngSpd_erpm : Inport  Port=6
  VDINR_HWAccelPedalPosn_pct : Inport  Port=7
  VDINR_EngTqMin_Nm : Inport  Port=8
  VDINR_EngTqMinValid_flg : Inport  Port=9
  VirtualPedalPosition : Subsystem  TreatAsAtomicUnit=on
  VTQEN_FinalAccelPedalPosn_pct : Outport
  wires:
  VDINR_EngTqMinValid_flg/1 -> VirtualPedalPosition/9(VDINR_EngTqMinValid_flg)
  VDINR_EngTqMin_Nm/1 -> VirtualPedalPosition/8(VDINR_EngTqMin_Nm)
  VTQEN_CruzEnblOn_flg/1 -> VirtualPedalPosition/7(VTQEN_CruzEnblOn_flg)
  VTQEN_VSGOVOn_flg/1 -> VirtualPedalPosition/6(VTQEN_VSGOVOn_flg)
  VTQEN_ECMTqSource_enum/1 -> VirtualPedalPosition/5(VTQEN_ECMTqSource_enum)
  VDINR_EngSpd_erpm/1 -> VirtualPedalPosition/4(VDINR_EngSpd_erpm)
  VDINR_HWAccelPedalPosn_pct/1 -> VirtualPedalPosition/3(VDINR_HWAccelPedalPosn_pct)
  VTQEN_EngBrakTqCap_Nm/1 -> VirtualPedalPosition/2(VTQEN_EngBrakTqCap_Nm)
  VirtualPedalPosition/1(VTQEN_FinalAccelPedalPosn_pct) -> VTQEN_FinalAccelPedalPosn_pct/1
  VTQEN_EngBrakTqReqFinal_Nm/1 -> VirtualPedalPosition/1(VTQEN_EngBrakTqReqFinal_Nm)

== system tqen/lib_divide5/Inter_Test ==
  u : Inport
  AND : Logic  AllPortsSameDT=off  OutDataTypeStr=boolean
  FixPt_Data_Type_Duplicate : S-Function  FunctionName=sfix_dtprop  Parameters=15,NumInputPorts  EnableBusSupport=off  mask(Data Type Duplicate){NumInputPorts=3}
      mask prompts: NumInputPorts "Number of input ports:"
      mask help: Force all inputs to have the exact same data type.
      mask Display: fprintf('Same\nDT')
  Lower_Limit : Constant  Value=lowlimit  OutDataTypeStr=Inherit: Inherit via back propagation
  Lower_Test : RelationalOperator  Operator=<=  OutDataTypeStr=fixdt(0, 8)  ZeroCross=off
  Upper_Limit : Constant  Value=uplimit  OutDataTypeStr=Inherit: Inherit via back propagation
  Upper_Test : RelationalOperator  Operator=<=  OutDataTypeStr=fixdt(0, 8)  ZeroCross=off
  y : Outport
  wires:
  AND/1 -> y/1
  u/1 -> Upper_Test/1, Lower_Test/2, FixPt_Data_Type_Duplicate/1
  Upper_Test/1 -> AND/2
  Lower_Test/1 -> AND/1
  Upper_Limit/1 -> FixPt_Data_Type_Duplicate/3, Upper_Test/2
  Lower_Limit/1 -> FixPt_Data_Type_Duplicate/2, Lower_Test/1

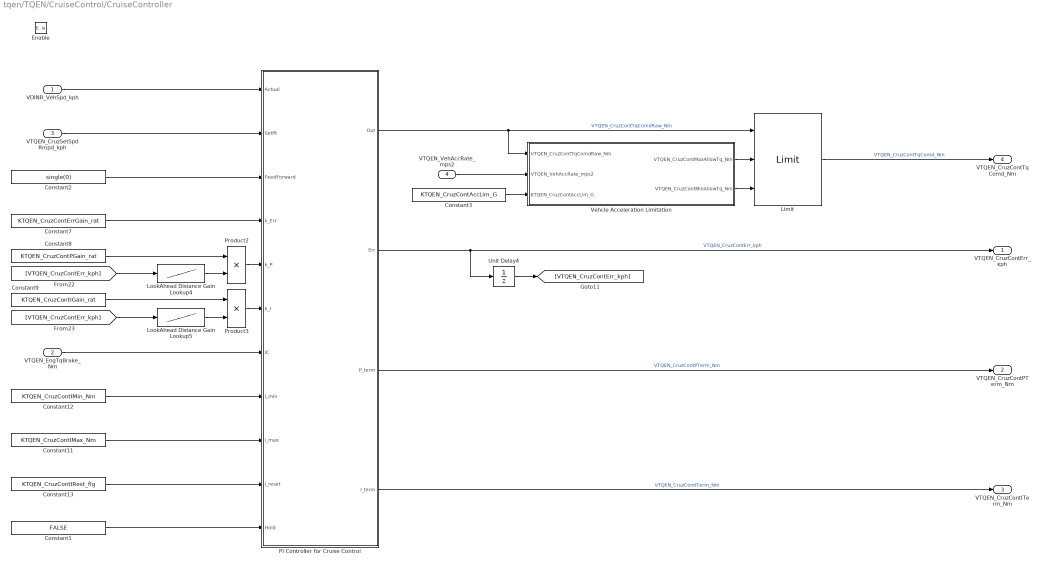
== system tqen/TQEN/CruiseControl/CruiseController ==
  VDINR_VehSpd_kph : Inport
  VTQEN_EngTqBrake_Nm : Inport  Port=2
  VTQEN_CruzSetSpdRmpd_kph : Inport  Port=3
  VTQEN_VehAccRate_mps2 : Inport  Port=4
  Enable : EnablePort  StatesWhenEnabling=reset
  Constant1 : Constant  Value=FALSE
  Constant11 : Constant  Value=KTQEN_CruzContIMax_Nm
  Constant12 : Constant  Value=KTQEN_CruzContIMin_Nm
  Constant13 : Constant  Value=KTQEN_CruzContIRest_flg
  Constant2 : Constant  Value=single(0)
  Constant3 : Constant  Value=KTQEN_CruzContAccLim_G
  Constant7 : Constant  Value=KTQEN_CruzContErrGain_rat
  Constant8 : Constant  Value=KTQEN_CruzContPGain_rat
  Constant9 : Constant  Value=KTQEN_CruzContIGain_rat
  Limit : hcu_lib/Limit  SystemSampleTime=-1
  LookAhead Distance Gain Lookup4 : Lookup  InputValues=ATQEN_CruzContPMult_X_kph  Table=MTQEN_CruzContPMult_rat  LookUpMeth=Interpolation-Use End Values
      settings: AttributesFormatString=%<InputValues>\n%<Table>
  LookAhead Distance Gain Lookup5 : Lookup  InputValues=ATQEN_CruzContIMult_X_kph  Table=MTQEN_CruzContIMult_rat  LookUpMeth=Interpolation-Use End Values
      settings: AttributesFormatString=%<InputValues>\n%<Table>
  PI Controller for Cruise Control : Subsystem  TreatAsAtomicUnit=on
  Product2 : Product  OutDataTypeStr=single  RndMeth=Zero
  Product3 : Product  OutDataTypeStr=single  RndMeth=Zero
  Unit Delay4 : UnitDelay  SampleTime=-1
  Vehcle Acceleration Limitation : Subsystem  TreatAsAtomicUnit=on
  VTQEN_CruzContErr_kph : Outport  OutputWhenDisabled=reset  InitialOutput=[0]
  VTQEN_CruzContPTerm_Nm : Outport  Port=2  OutputWhenDisabled=reset  InitialOutput=[0]
  VTQEN_CruzContITerm_Nm : Outport  Port=3  OutputWhenDisabled=reset  InitialOutput=[0]
  VTQEN_CruzContTqComd_Nm : Outport  Port=4  OutputWhenDisabled=reset  InitialOutput=[0]
  wires:
  Vehcle Acceleration Limitation/2(VTQEN_CruzContMinAllowTq_Nm) -> Limit/3
  Vehcle Acceleration Limitation/1(VTQEN_CruzContMaxAllowTq_Nm) -> Limit/2
  Constant2/1 -> PI Controller for Cruise Control/3(FeedForward)
  Constant1/1 -> PI Controller for Cruise Control/11(Hold)
  Unit Delay4/1 -> [VTQEN_CruzContErr_kph]
  [VTQEN_CruzContErr_kph] -> LookAhead Distance Gain Lookup5/1
  Constant9/1 -> Product3/1
  Product3/1 -> PI Controller for Cruise Control/6(k_I)
  LookAhead Distance Gain Lookup5/1 -> Product3/2
  [VTQEN_CruzContErr_kph] -> LookAhead Distance Gain Lookup4/1
  LookAhead Distance Gain Lookup4/1 -> Product2/2
  Product2/1 -> PI Controller for Cruise Control/5(k_P)
  PI Controller for Cruise Control/4(I_term) -> VTQEN_CruzContITerm_Nm/1  "VTQEN_CruzContITerm_Nm"
  PI Controller for Cruise Control/3(P_term) -> VTQEN_CruzContPTerm_Nm/1  "VTQEN_CruzContPTerm_Nm"
  PI Controller for Cruise Control/2(Err) -> VTQEN_CruzContErr_kph/1, Unit Delay4/1  "VTQEN_CruzContErr_kph"
  Constant13/1 -> PI Controller for Cruise Control/10(I_reset)
  Constant11/1 -> PI Controller for Cruise Control/9(I_max)
  Constant12/1 -> PI Controller for Cruise Control/8(I_min)
  VTQEN_EngTqBrake_Nm/1 -> PI Controller for Cruise Control/7(IC)
  Constant8/1 -> Product2/1
  Constant7/1 -> PI Controller for Cruise Control/4(k_Err)
  VTQEN_CruzSetSpdRmpd_kph/1 -> PI Controller for Cruise Control/2(SetPt)
  VDINR_VehSpd_kph/1 -> PI Controller for Cruise Control/1(Actual)
  Constant3/1 -> Vehcle Acceleration Limitation/3(KTQEN_CruzContAccLim_G)
  VTQEN_VehAccRate_mps2/1 -> Vehcle Acceleration Limitation/2(VTQEN_VehAccRate_mps2)
  Limit/1 -> VTQEN_CruzContTqComd_Nm/1  "VTQEN_CruzContTqComd_Nm"
  PI Controller for Cruise Control/1(Out) -> Limit/1, Vehcle Acceleration Limitation/1(VTQEN_CruzContTqComdRaw_Nm)  "VTQEN_CruzContTqComdRaw_Nm"

== system tqen/TQEN/CruiseControl/Rate_Limit ==
  Data_Input : Inport
  Initial_condition : Inport  Port=2
  Rising_Rate : Inport  Port=3
  Falling_Rate : Inport  Port=4
  Enable : EnablePort  StatesWhenEnabling=reset
  RateLimiter : Subsystem
  Data_Output : Outport  OutputWhenDisabled=reset  InitialOutput=[0]
  wires:
  Rising_Rate/1 -> RateLimiter/2(Rising Rate)
  Falling_Rate/1 -> RateLimiter/3(Falling Rate)
  Initial_condition/1 -> RateLimiter/4(Initial_Condition)
  Data_Input/1 -> RateLimiter/1(Data_Input)
  RateLimiter/1(Data_Output) -> Data_Output/1

== system tqen/TQEN/CruiseControl/Trigger signal generator ==
  Constant3 : Constant  Value=KTQEN_VehAccCalRate_s
  trigger signal generator : Subsystem  TreatAsAtomicUnit=on
  Trigger_signal : Outport
  wires:
  trigger signal generator/1(Trigger_signal) -> Trigger_signal/1
  Constant3/1 -> trigger signal generator/1(Time_dur [s])

== system tqen/TQEN/CruiseControl/Vehicle Acceleration Calculation ==
  note: m/s^2
  note: m/s
  note: km/h
  In1 : Inport
  Trigger : TriggerPort
  Constant2 : Constant  Value=KTQEN_VehAccCalRate_s
  Constant4 : Constant  Value=KTQEN_VehAccFltConst_s
  Constant5 : Constant  Value=KTQEN_VehAccCalRate_s
  Divide : Product  Inputs=*/
  Gain : Gain  Gain=1000/3600
  Gain1 : Gain  Gain=1/9.81  OutDataTypeStr=single
  Sum : Sum  Inputs=+-
  Terminator1 : Terminator
  Unit Delay : UnitDelay  SampleTime=-1
  signal_filter : Subsystem
  Out1 : Outport
  wires:
  Gain1/1 -> Terminator1/1  "VTQEN_VehAccRate_g"
  signal_filter/1(raw_input_filt) -> Gain1/1, Out1/1  "VTQEN_VehAccRate_mps2"
  Constant5/1 -> Divide/2
  Gain/1 -> Divide/1
  Sum/1 -> Gain/1
  Unit Delay/1 -> Sum/2
  In1/1 -> Sum/1, Unit Delay/1
  Constant2/1 -> signal_filter/3(Ts)
  Constant4/1 -> signal_filter/2(Tc)
  Divide/1 -> signal_filter/1(raw_input)  "VTQEN_VehAccRateUnFlt_mps2"

== system tqen/TQEN/ExternalTorqueDemand/Timer2 ==
  Enable : EnablePort  StatesWhenEnabling=reset  ZeroCross=off
  Constant : Constant  Value=C_TICK_TIME_S
  Sum : Sum  Inputs=|++  SaturateOnIntegerOverflow=on  InputSameDT=on
  Unit Delay : UnitDelay  SampleTime=-1
  Timer (sec) : Outport  OutputWhenDisabled=reset  InitialOutput=0
  wires:
  Constant/1 -> Sum/1
  Sum/1 -> Unit Delay/1
  Unit Delay/1 -> Sum/2, Timer (sec)/1

== system tqen/TQEN/Governor/Governor ==
  VTQEN_VSGOVOn_flg : Inport
  VTQEN_VSGOVTqComdFinal_Nm : Inport  Port=2
  VDINR_ADASVehSpdLimReqValid_flg : Inport  Port=3
  VDINR_NowGearPosn_enum : Inport  Port=4
  VDINR_VehSpdValid_flg : Inport  Port=5
  VDINR_VehSpd_kph : Inport  Port=6
  Constant : Constant  Value=ENUM_GEARPOSN_PN
  Constant1 : Constant  Value=single(10000)
  Constant2 : Constant  Value=KTQEN_VSGOVMinVehSpd_kph
  Logical Operator1 : Logic  Inputs=5  AllPortsSameDT=off  OutDataTypeStr=boolean
  Relational Operator : RelationalOperator  Operator=~=  OutDataTypeStr=boolean
  Relational Operator2 : RelationalOperator  Operator=>  OutDataTypeStr=boolean
  Switch2 : Switch  Criteria=u2 ~= 0
  VTQEN_VSGOVTqBound_Nm : Outport
  wires:
  VDINR_ADASVehSpdLimReqValid_flg/1 -> Logical Operator1/3
  Constant2/1 -> Relational Operator2/2
  Constant/1 -> Relational Operator/2
  VTQEN_VSGOVOn_flg/1 -> Logical Operator1/1
  VDINR_NowGearPosn_enum/1 -> Relational Operator/1
  VDINR_VehSpdValid_flg/1 -> Logical Operator1/2
  Relational Operator/1 -> Logical Operator1/4
  VDINR_VehSpd_kph/1 -> Relational Operator2/1
  Relational Operator2/1 -> Logical Operator1/5
  Logical Operator1/1 -> Switch2/2
  VTQEN_VSGOVTqComdFinal_Nm/1 -> Switch2/1
  Constant1/1 -> Switch2/3
  Switch2/1 -> VTQEN_VSGOVTqBound_Nm/1  "VTQEN_VSGOVTqBound_Nm"

== system tqen/TQEN/Governor/Max_Min_Brake_Torque ==
  Constant1 : Constant  Value=KTQEN_EngBrkTqMaxOvrd_Nm
  Constant4 : Constant  Value=KTQEN_EngBrkTqMinOvrd_Nm
  VTQEN_EngBrkTqReqMax_Nm : Outport
  VTQEN_EngBrakTqReqMin_Nm : Outport  Port=2
  wires:
  Constant1/1 -> VTQEN_EngBrkTqReqMax_Nm/1  "VTQEN_EngBrakTqReqMax_Nm"
  Constant4/1 -> VTQEN_EngBrakTqReqMin_Nm/1  "VTQEN_EngBrakTqReqMin_Nm"

== system tqen/TQEN/Governor/TorqueSourceDetermination ==
  VTQEN_EngBrakTqReqGoverd_Nm : Inport
  VTQEN_VSGOVTqBound_Nm : Inport  Port=2
  VDINR_ADASPTTqReqApplable_flg : Inport  Port=3
  VDINR_BrkLampOn_flg : Inport  Port=4
  VTQEN_ExternalTqDemLim_flg : Inport  Port=5
  Constant : Constant  Value=ENUM_ECMTQSOURCE_INTERNAL
  Constant1 : Constant  Value=ENUM_ECMTQSOURCE_EXTERNAL
  Constant2 : Constant  Value=ENUM_ECMTQSOURCE_TORQUELIM
  Logical Operator : Logic  Operator=OR  Inputs=3  AllPortsSameDT=off  OutDataTypeStr=boolean
  Relational Operator : RelationalOperator  Operator===  OutDataTypeStr=boolean
  Switch1 : Switch  Criteria=u2 ~= 0
  Switch2 : Switch  Criteria=u2 ~= 0
  VTQEN_ECMTqSource_enum : Outport
  wires:
  Logical Operator/1 -> Switch1/2
  VDINR_BrkLampOn_flg/1 -> Logical Operator/3
  VTQEN_ExternalTqDemLim_flg/1 -> Logical Operator/1
  Constant2/1 -> Switch1/1
  Switch2/1 -> Switch1/3
  Relational Operator/1 -> Logical Operator/2
  VTQEN_VSGOVTqBound_Nm/1 -> Relational Operator/2
  VTQEN_EngBrakTqReqGoverd_Nm/1 -> Relational Operator/1
  VDINR_ADASPTTqReqApplable_flg/1 -> Switch2/2
  Constant1/1 -> Switch2/1
  Constant/1 -> Switch2/3
  Switch1/1 -> VTQEN_ECMTqSource_enum/1  "VTQEN_ECMTqSource_enum"

== system tqen/TQEN/Governor/Torque_Limitation ==
  VTQEN_EngBrkTqReqMax_Nm : Inport  OutDataTypeStr=single
  VTQEN_EngBrakTqReqMin_Nm : Inport  Port=2  OutDataTypeStr=single
  VTQEN_EngBrakTqReqGoverd_Nm : Inport  Port=3  OutDataTypeStr=single
  Limit3 : tqen/Limit3  SystemSampleTime=-1
  VTQEN_EngBrakTqReqFinal_Nm : Outport
  wires:
  VTQEN_EngBrakTqReqMin_Nm/1 -> Limit3/3
  VTQEN_EngBrkTqReqMax_Nm/1 -> Limit3/2
  VTQEN_EngBrakTqReqGoverd_Nm/1 -> Limit3/1
  Limit3/1 -> VTQEN_EngBrakTqReqFinal_Nm/1  "VTQEN_EngBrakTqReqFinal_Nm"

== system tqen/TQEN/Governor/Vehcle Speed Governing ==
  note: 0=Pedal
      | 1=External
      | 2=Governing
  VTQEN_ECMTqSource_enum : Inport
  VDINR_VehSpd_kph : Inport  Port=2
  VTQEN_EngBrakTqReqRaw_Nm : Inport  Port=3
  VDINR_ADASVehSpdLimReq_kph : Inport  Port=4
  Constant1 : Constant  Value=KTQEN_VehSpdMaxVal_kph
  Constant2 : Constant  Value=KTQEN_VSGOVTqDefault_Nm
  Governing State Determination : Stateflow chart  TreatAsAtomicUnit=on
  MinMax : MinMax  Inputs=2
  Switch : Switch  Criteria=u2 ~= 0
  Terminator : Terminator
  Terminator1 : Terminator
  Terminator2 : Terminator
  Vehicle Speed Governor : Subsystem  TreatAsAtomicUnit=on
  VTQEN_VSGOVOn_flg : Outport
  VTQEN_VSGOVTqComdFinal_Nm : Outport  Port=2
  wires:
  VDINR_ADASVehSpdLimReq_kph/1 -> MinMax/2
  Constant1/1 -> MinMax/1
  MinMax/1 -> [VTQEN_VehSpdLimVal_kph], Governing State Determination/1(VTQEN_VehSpdLimVal_kph)  "VTQEN_VehSpdLimVal_kph"
  VDINR_VehSpd_kph/1 -> [VDINR_VehSpd_kph], Governing State Determination/2(VDINR_VehSpd_kph)
  VTQEN_ECMTqSource_enum/1 -> Governing State Determination/3(VTQEN_EngTqSource_enum)
  Governing State Determination/1(VTQEN_VSGOVOn_flg) -> VTQEN_VSGOVOn_flg/1, Switch/2, Vehicle Speed Governor/Enable
  Constant2/1 -> Switch/3
  Vehicle Speed Governor/4(VTQEN_VSGOVTqComd_Nm) -> Switch/1
  [VDINR_VehSpd_kph] -> Vehicle Speed Governor/1(VDINR_VehSpd_kph)
  VTQEN_EngBrakTqReqRaw_Nm/1 -> Vehicle Speed Governor/2(VTQEN_EngBrakTqReqRaw_Nm)
  [VTQEN_VehSpdLimVal_kph] -> Vehicle Speed Governor/3(VTQEN_VehSpdLimVal_kph)
  Switch/1 -> VTQEN_VSGOVTqComdFinal_Nm/1  "VTQEN_VSGOVTqComdFinal_Nm"
  Vehicle Speed Governor/1(VTQEN_VSGOVErr_kph) -> Terminator/1
  Vehicle Speed Governor/2(VTQEN_VSGOVPTerm_Nm) -> Terminator1/1
  Vehicle Speed Governor/3(VTQEN_VSGOVITerm_Nm) -> Terminator2/1

== system tqen/TQEN/MaximumAllowableBrakeTorque/EngTqCapacity ==
  VDINR_EngTqMax_Nm : Inport
  VDINR_EngTqMin_Nm : Inport  Port=2
  VDINR_EngTqMinValid_flg : Inport  Port=3
  VDINR_EngTqMaxValid_flg : Inport  Port=4
  VDINR_EngSpd_erpm : Inport  Port=5
  Add : Sum  Inputs=+-
  Logical Operator : Logic  AllPortsSameDT=off  OutDataTypeStr=boolean
  Lookup Table : Lookup  InputValues=ATQEN_EngTqBrkMap_X_erpm  Table=MTQEN_EngTqBrkMap_Y_Nm  LookUpMeth=Interpolation-Use End Values
      settings: AttributesFormatString=<input =%<InputValues>>\n<output = %<Table>>
  Switch : Switch  Criteria=u2 ~= 0
  VTQEN_EngBrakTqCap_Nm : Outport
  wires:
  Add/1 -> Switch/1
  VDINR_EngSpd_erpm/1 -> Lookup Table/1
  VDINR_EngTqMaxValid_flg/1 -> Logical Operator/2
  Switch/1 -> VTQEN_EngBrakTqCap_Nm/1  "VTQEN_EngBrakTqCap_Nm"
  VDINR_EngTqMinValid_flg/1 -> Logical Operator/1
  VDINR_EngTqMin_Nm/1 -> Add/2
  VDINR_EngTqMax_Nm/1 -> Add/1
  Lookup Table/1 -> Switch/3
  Logical Operator/1 -> Switch/2

== system tqen/TQEN/MaximumEngineIndicatedTorque/Max_Indicated_Torque ==
  VDINR_EngTqFriction_Nm : Inport
  Add : Sum
  Constant1 : Constant  Value=KTQEN_EngBrkTqMaxOvrd_Nm
  VTQEN_EngIndTqReqMax_Nm : Outport
  wires:
  Constant1/1 -> Add/1
  VDINR_EngTqFriction_Nm/1 -> Add/2
  Add/1 -> VTQEN_EngIndTqReqMax_Nm/1  "VTQEN_EngIndTqReqMax_Nm"

== system tqen/TQEN/PedalTorqueDemand/PedalTorqueDemandCalculation ==
  task_time_s : Inport
  VDINR_HWAccelPedalPosn_pct : Inport  Port=2
  VDINR_EngSpd_erpm : Inport  Port=3
  VDINR_VehSpd_kph : Inport  Port=4
  VDINR_BrkLampOn_flg : Inport  Port=5
  VTQEN_EngBrakTqCap_Nm : Inport  Port=6
  PedalFeelMap : Subsystem
  PedalTorqueCalculation : Subsystem
  VTQEN_PedalTqDem_Nm : Outport
  wires:
  PedalFeelMap/2(VTQEN_PedalTqSportlHiD_pct) -> PedalTorqueCalculation/4(VTQEN_PedalTqSportlHiD_pct)
  PedalFeelMap/1(VTQEN_PedalTqSportLoD_pct) -> PedalTorqueCalculation/3(VTQEN_PedalTqSportLoD_pct)
  VTQEN_EngBrakTqCap_Nm/1 -> PedalTorqueCalculation/6(VTQEN_EngBrakTqCap_Nm)
  VDINR_VehSpd_kph/1 -> PedalTorqueCalculation/5(VDINR_VehSpd_kph)
  VDINR_EngSpd_erpm/1 -> PedalFeelMap/2(VDINR_EngSpd_erpm)
  VDINR_HWAccelPedalPosn_pct/1 -> PedalFeelMap/1(VDINR_HWAccelPedalPosn_pct), PedalTorqueCalculation/2(VDINR_HWAccelPedalPosn_pct)
  PedalTorqueCalculation/1(VTQEN_PedalTqDem_Nm) -> VTQEN_PedalTqDem_Nm/1
  VDINR_BrkLampOn_flg/1 -> PedalTorqueCalculation/7(VDINR_BrkLampOn_flg)
  task_time_s/1 -> PedalTorqueCalculation/1(task_time_s)
